simulink model "Copter_System_discrete_sfun"  (Simulink 7.4)
settings: Solver=FixedStepDiscrete  StartTime=0.0  StopTime=tend  FixedStep=Ts  RelTol=1e-3
values from neighbouring files (symbols this model uses):
  f1 = (I_y-I_z)/I_x    [quadrocopter_param.m]
  f2 = rot.J_z/I_x    [quadrocopter_param.m]
  f3 = (I_z-I_x)/I_y    [quadrocopter_param.m]
  f4 = rot.J_z/I_y    [quadrocopter_param.m]
  f5 = (I_x-I_y)/I_z    [quadrocopter_param.m]
  g = 9.81    [complementary_filter_param.m]    (also in quadrocopter_param.m)
  I_x = elec.I_x+bat.I_x+2*boom.I_1x+2*boom.I_1y+2*mot.I_1x+2*mot.I_1y+                             2*rot.I_1x+2*rot.I_1y    [quadrocopter_param.m]
  I_y = elec.I_y+bat.I_y+2*boom.I_1x+2*boom.I_1y+2*mot.I_1x+2*mot.I_1y+                             2*rot.I_1x+2*rot.I_1y    [quadrocopter_param.m]
  I_z = elec.I_z+bat.I_z+4*boom.I_1z+4*mot.I_1z+4*rot.I_1z    [quadrocopter_param.m]
  m = elec.m+bat.m+boom.m+(4*mot.m)+(4*rot.m)    [quadrocopter_param.m]
  shift = 1000    [quadrocopter_param.m]
  speed = rpm.*(2*pi/60)    [quadrocopter_param.m]
  thrust = [0.58 1 1.33 2 2.54 3.33 4.08 4.54]    [quadrocopter_param.m]
  Ts = 0.01    [complementary_filter_param.m]    (also in quadrocopter_param.m)
undefined symbols (not defined in the file or in its folder): boom, DiscIntNeverNeededParam
libraries: simulink x4, dspinverses x1
settings Model: Creator=Sreekanth  LastModifiedBy=Sreekanth
settings DebuggingCC: ArtificialAlgebraicLoopMsg=none

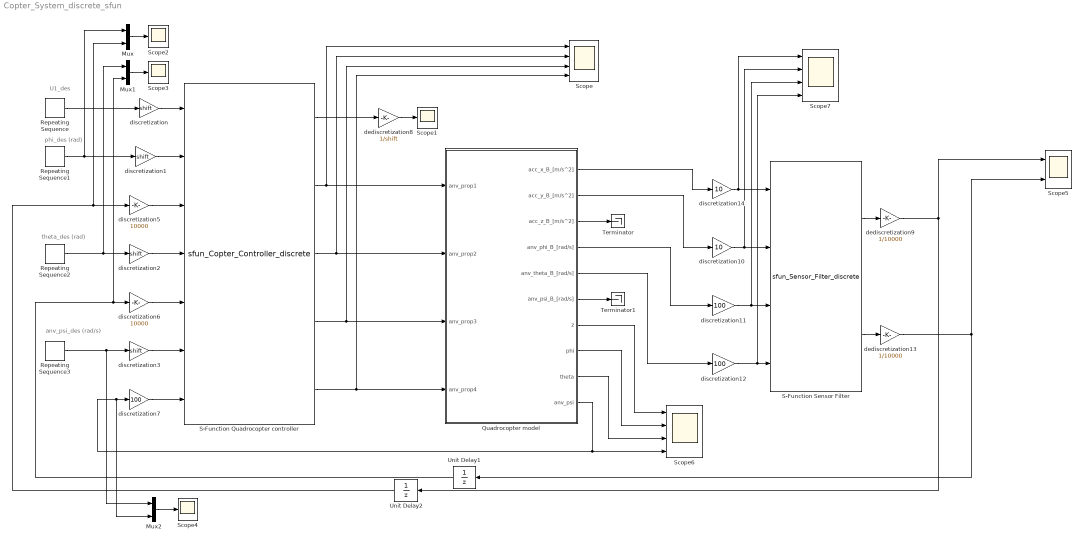
== system Copter_System_discrete_sfun ==
  note: U1_des
  note: phi_des (rad)
  note: theta_des (rad)
  note: anv_psi_des (rad/s)
  Mux : Mux  Inputs=2
  Mux1 : Mux  Inputs=2
  Mux2 : Mux  Inputs=2
  Quadrocopter model : Subsystem
  Repeating Sequence : simulink/Sources/Repeating Sequence  SystemSampleTime=-1  rep_seq_t=desforce.time  rep_seq_y=desforce.force
  Repeating Sequence1 : simulink/Sources/Repeating Sequence  SystemSampleTime=-1  rep_seq_t=desroll.time  rep_seq_y=desroll.angle
  Repeating Sequence2 : simulink/Sources/Repeating Sequence  SystemSampleTime=-1  rep_seq_t=despitch.time  rep_seq_y=despitch.angle
  Repeating Sequence3 : simulink/Sources/Repeating Sequence  SystemSampleTime=-1  rep_seq_t=desyaw.time  rep_seq_y=desyaw.velocity
  S-Function Quadrocopter controller : S-Function  FunctionName=sfun_Copter_Controller_discrete  Parameters=[8 4 8 8 4 8 8 3 1]  EnableBusSupport=off
      mask Display:
      | port_label('input',1,'U1_des')
      | port_label('input',2,'phi_des')
      | port_label('input',3,'phi_filt')
      | port_label('input',4,'theta_des')
      | port_label('input',5,'theta_filt')
      | port_label('input',6,'anv_psi_des')
      | port_label('input',7,'anv_psi')
      | port_label('output',1,'U1_out')
      | port_label('output',2,'anv_prop1')
      | port_label('output',3,'anv_prop2')
      | port_label('output',4,'anv_prop3')
      | port_label('output',5,'anv_prop4')
  S-Function Sensor Filter : S-Function  FunctionName=sfun_Sensor_Filter_discrete  EnableBusSupport=off
      mask Display:
      | port_label('input',1,'acc_x_B')
      | port_label('input',2,'acc_y_B')
      | port_label('input',3,'anv_phi_B')
      | port_label('input',4,'anv_theta_B')
      | port_label('output',1,'phi_filt')
      | port_label('output',2,'theta_filt')
  Scope : Scope  NumInputPorts=4
      settings: TimeRange=30  YMin=0~0~0~0  YMax=6000~6000~6000~6000
  Scope{1..4} (4 alike) : Scope
      Scope1 settings: YMax=20
      Scope2 settings: TimeRange=30  YMin=0  YMax=0.275  SaveName=ScopeData2
      Scope3 settings: TimeRange=30  YMin=0  YMax=0.275  SaveName=ScopeData14
      Scope4 settings: TimeRange=30  YMin=-0.02  YMax=0.3  SaveName=ScopeData15
  Scope5 : Scope  NumInputPorts=2
      settings: YMin=-5~-5  YMax=5~5  SaveName=ScopeData12
  Scope6 : Scope  NumInputPorts=4
      settings: TimeRange=30  YMin=-5~-5~-5~-5  YMax=5~5~5~5  SaveName=ScopeData13
  Scope7 : Scope  NumInputPorts=4
      settings: TimeRange=30  YMin=-5~-5~-5~-5  YMax=5~5~5~5  SaveName=ScopeData16
  Terminator : Terminator
  Terminator1 : Terminator
  Unit Delay1 : UnitDelay  SampleTime=-1
  Unit Delay2 : UnitDelay  SampleTime=-1
  dediscretization13 : Gain  Gain=1/10000  ParameterDataType=fixdt(1, 16)  ParameterScaling=2^0  OutDataTypeMode=double  OutDataType=fixdt(1, 16)  OutScaling=2^0  OutDataTypeStr=double
  dediscretization8 : Gain  Gain=1/shift  ParameterDataType=fixdt(1, 16)  ParameterScaling=2^0  OutDataTypeMode=double  OutDataType=fixdt(1, 16)  OutScaling=2^0  OutDataTypeStr=double
  dediscretization9 : Gain  Gain=1/10000  ParameterDataType=fixdt(1, 16)  ParameterScaling=2^0  OutDataTypeMode=double  OutDataType=fixdt(1, 16)  OutScaling=2^0  OutDataTypeStr=double
  discretization{,1..3} (4 alike) : Gain  Gain=shift  ParameterDataType=fixdt(1, 16)  ParameterScaling=2^0  OutDataTypeMode=int16  OutDataType=fixdt(1, 16)  OutScaling=2^0  OutDataTypeStr=int16
  discretization10 : Gain  Gain=10  ParameterDataType=fixdt(1, 16)  ParameterScaling=2^0  OutDataTypeMode=int16  OutDataType=fixdt(1, 16)  OutScaling=2^0  OutDataTypeStr=int16
  discretization11 : Gain  Gain=100  ParameterDataType=fixdt(1, 16)  ParameterScaling=2^0  OutDataTypeMode=int16  OutDataType=fixdt(1, 16)  OutScaling=2^0  OutDataTypeStr=int16
  discretization12 : Gain  Gain=100  ParameterDataType=fixdt(1, 16)  ParameterScaling=2^0  OutDataTypeMode=int16  OutDataType=fixdt(1, 16)  OutScaling=2^0  OutDataTypeStr=int16
  discretization14 : Gain  Gain=10  ParameterDataType=fixdt(1, 16)  ParameterScaling=2^0  OutDataTypeMode=int16  OutDataType=fixdt(1, 16)  OutScaling=2^0  OutDataTypeStr=int16
  discretization5 : Gain  Gain=10000  ParameterDataType=fixdt(1, 16)  ParameterScaling=2^0  OutDataTypeMode=int16  OutDataType=fixdt(1, 16)  OutScaling=2^0  OutDataTypeStr=int16
  discretization6 : Gain  Gain=10000  ParameterDataType=fixdt(1, 16)  ParameterScaling=2^0  OutDataTypeMode=int16  OutDataType=fixdt(1, 16)  OutScaling=2^0  OutDataTypeStr=int16
  discretization7 : Gain  Gain=100  ParameterDataType=fixdt(1, 16)  ParameterScaling=2^0  OutDataTypeMode=int16  OutDataType=fixdt(1, 16)  OutScaling=2^0  OutDataTypeStr=int16
  wires:
  Repeating Sequence/1 -> discretization/1
  discretization/1 -> S-Function Quadrocopter controller/1
  Repeating Sequence1/1 -> discretization1/1, Mux/1
  discretization1/1 -> S-Function Quadrocopter controller/2
  Repeating Sequence2/1 -> discretization2/1, Mux1/1
  discretization2/1 -> S-Function Quadrocopter controller/4
  Repeating Sequence3/1 -> discretization3/1, Mux2/1
  discretization3/1 -> S-Function Quadrocopter controller/6
  discretization5/1 -> S-Function Quadrocopter controller/3
  discretization6/1 -> S-Function Quadrocopter controller/5
  discretization7/1 -> S-Function Quadrocopter controller/7
  S-Function Quadrocopter controller/1 -> dediscretization8/1
  S-Function Quadrocopter controller/2 -> Scope/1, Quadrocopter model/1(anv_prop1)
  S-Function Quadrocopter controller/3 -> Scope/2, Quadrocopter model/2(anv_prop2)
  S-Function Quadrocopter controller/4 -> Scope/3, Quadrocopter model/3(anv_prop3)
  S-Function Quadrocopter controller/5 -> Scope/4, Quadrocopter model/4(anv_prop4)
  dediscretization8/1 -> Scope1/1
  Quadrocopter model/3(acc_z_B_[m/s^2]) -> Terminator/1
  Quadrocopter model/6(anv_psi_B_[rad/s]) -> Terminator1/1
  discretization14/1 -> S-Function Sensor Filter/1, Scope7/1
  discretization10/1 -> S-Function Sensor Filter/2, Scope7/2
  discretization11/1 -> S-Function Sensor Filter/3, Scope7/3
  discretization12/1 -> S-Function Sensor Filter/4, Scope7/4
  S-Function Sensor Filter/1 -> dediscretization9/1
  S-Function Sensor Filter/2 -> dediscretization13/1
  dediscretization9/1 -> Scope5/1, Unit Delay2/1
  Quadrocopter model/1(acc_x_B_[m/s^2]) -> discretization14/1
  Quadrocopter model/2(acc_y_B_[m/s^2]) -> discretization10/1
  Quadrocopter model/4(anv_phi_B_[rad/s]) -> discretization11/1
  Quadrocopter model/5(anv_theta_B_[rad/s]) -> discretization12/1
  dediscretization13/1 -> Scope5/2, Unit Delay1/1
  Quadrocopter model/10(anv_psi) -> Scope6/4, discretization7/1, Mux2/2
  Unit Delay1/1 -> discretization6/1, Mux1/2
  Unit Delay2/1 -> discretization5/1, Mux/2
  Mux/1 -> Scope2/1
  Mux1/1 -> Scope3/1
  Mux2/1 -> Scope4/1
  Quadrocopter model/7(z) -> Scope6/1
  Quadrocopter model/8(phi) -> Scope6/2
  Quadrocopter model/9(theta) -> Scope6/3

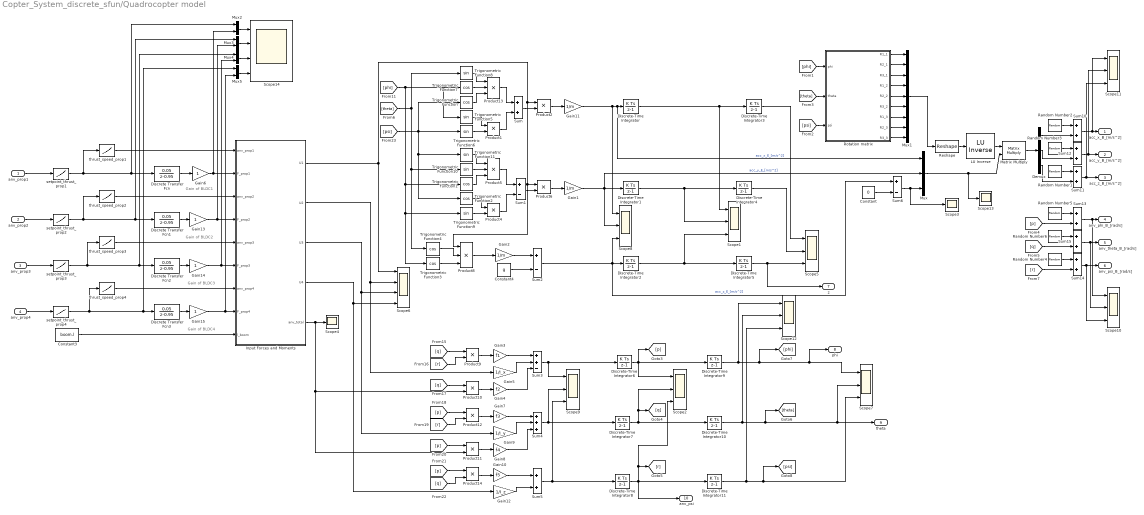
== system Copter_System_discrete_sfun/Quadrocopter model ==
  note: Gain of BLDC1
  note: Gain of BLDC2
  note: Gain of BLDC3
  note: Gain of BLDC4
  anv_prop1 : Inport  OutDataType=fixdt(1, 16)  OutScaling=2^0
  anv_prop2 : Inport  Port=2  OutDataType=fixdt(1, 16)  OutScaling=2^0
  anv_prop3 : Inport  Port=3  OutDataType=fixdt(1, 16)  OutScaling=2^0
  anv_prop4 : Inport  Port=4  OutDataType=fixdt(1, 16)  OutScaling=2^0
  " LU Inverse" : dspinverses/ LU Inverse  SystemSampleTime=-1
  Constant : Constant  Value=0  OutDataType=fixdt(1, 16)  OutScaling=2^0  SampleTime=Ts
  Constant3 : Constant  Value=boom.l  OutDataType=fixdt(1, 16)  OutScaling=2^0
  Constant4 : Constant  Value=g  OutDataType=fixdt(1, 16)  OutScaling=2^0  SampleTime=Ts
  Demux : Demux  Outputs=3
  Discrete Transfer Fcn{,1..3} (4 alike) : DiscreteTransferFcn  Numerator=[0.05]  Denominator=[1 -0.95]  SampleTime=Ts  OutDataTypeStr=int16
  Discrete-Time Integrator{,1..11} (12 alike) : DiscreteIntegrator  SampleTime=Ts  OutDataType=fixdt(1, 16)  OutScaling=2^0  ICPrevOutput=DiscIntNeverNeededParam  ICPrevScaledInput=DiscIntNeverNeededParam
  Gain1 : Gain  Gain=1/m  ParameterDataType=fixdt(1, 16)  ParameterScaling=2^0  OutDataType=fixdt(1, 16)  OutScaling=2^0
  Gain10 : Gain  Gain=f5  ParameterDataType=fixdt(1, 16)  ParameterScaling=2^0  OutDataType=fixdt(1, 16)  OutScaling=2^0
  Gain11 : Gain  Gain=1/m  ParameterDataType=fixdt(1, 16)  ParameterScaling=2^0  OutDataType=fixdt(1, 16)  OutScaling=2^0
  Gain12 : Gain  Gain=1/I_z  ParameterDataType=fixdt(1, 16)  ParameterScaling=2^0  OutDataType=fixdt(1, 16)  OutScaling=2^0
  Gain{6,13..15} (4 alike) : Gain  ParameterDataType=fixdt(1, 16)  ParameterScaling=2^0  OutDataTypeMode=double  OutDataType=fixdt(1, 16)  OutScaling=2^0  OutDataTypeStr=double
  Gain2 : Gain  Gain=1/m  ParameterDataType=fixdt(1, 16)  ParameterScaling=2^0  OutDataType=fixdt(1, 16)  OutScaling=2^0
  Gain3 : Gain  Gain=f1  ParameterDataType=fixdt(1, 16)  ParameterScaling=2^0  OutDataType=fixdt(1, 16)  OutScaling=2^0
  Gain4 : Gain  Gain=f2  ParameterDataType=fixdt(1, 16)  ParameterScaling=2^0  OutDataType=fixdt(1, 16)  OutScaling=2^0
  Gain5 : Gain  Gain=1/I_x  ParameterDataType=fixdt(1, 16)  ParameterScaling=2^0  OutDataType=fixdt(1, 16)  OutScaling=2^0
  Gain7 : Gain  Gain=f3  ParameterDataType=fixdt(1, 16)  ParameterScaling=2^0  OutDataType=fixdt(1, 16)  OutScaling=2^0
  Gain8 : Gain  Gain=f4  ParameterDataType=fixdt(1, 16)  ParameterScaling=2^0  OutDataType=fixdt(1, 16)  OutScaling=2^0
  Gain9 : Gain  Gain=1/I_y  ParameterDataType=fixdt(1, 16)  ParameterScaling=2^0  OutDataType=fixdt(1, 16)  OutScaling=2^0
  Input Forces and Moments : Stateflow chart
  Matrix Multiply : Product  Multiplication=Matrix(*)  OutDataType=sfix(16)  OutScaling=2^0
  Mux : Mux  Inputs=3
  Mux1 : Mux  Inputs=9
  Mux{2..5} (4 alike) : Mux  Inputs=2
  Product{1..2,4,6,9..12,14} (9 alike) : Product  OutDataType=fixdt(1, 16)  OutScaling=2^0  RndMeth=Zero
  Product13 : Product  Inputs=3  OutDataType=fixdt(1, 16)  OutScaling=2^0  RndMeth=Zero
  Product5 : Product  Inputs=3  OutDataType=fixdt(1, 16)  OutScaling=2^0  RndMeth=Zero
  Product8 : Product  Inputs=3  OutDataType=fixdt(1, 16)  OutScaling=2^0  RndMeth=Zero
  Random Number{1..6} (6 alike) : RandomNumber  Variance=0  SampleTime=Ts
  Reshape : Reshape  OutputDimensionality=Customize  OutputDimensions=[3,3]
  Rotation matrix : Stateflow chart
  Scope{1..2,5,7..12} (9 alike) : Scope  NumInputPorts=3
      Scope1 settings: YMin=-5~-5~-5  YMax=5~5~5  SaveName=ScopeData21
      Scope10 settings: YMin=-5~-5~-5  YMax=5~5~5  SaveName=ScopeData9
      Scope11 settings: YMin=-5~-5~-5  YMax=5~5~5  SaveName=ScopeData10
      Scope12 settings: YMin=-5~-5~-5  YMax=5~5~5  SaveName=ScopeData11
      Scope2 settings: YMin=-5~-5~-5  YMax=5~5~5  SaveName=ScopeData24
      Scope5 settings: YMin=-5~-5~-5  YMax=5~5~5  SaveName=ScopeData3
      Scope7 settings: TimeRange=30  YMin=-0.05~-0.2~-0.5  YMax=0.3~0.15~3  SaveName=ScopeData6
      Scope8 settings: TimeRange=30  YMin=-1~-1~3  YMax=1~1~10  SaveName=ScopeData7
      Scope9 settings: YMin=-5~-5~-5  YMax=5~5~5  SaveName=ScopeData8
  Scope13 : Scope
      settings: SaveName=ScopeData22
  Scope14 : Scope  NumInputPorts=4
      settings: YMin=-5~-5~-5~-5  YMax=5~5~5~5  SaveName=ScopeData23
  Scope3 : Scope
      settings: SaveName=ScopeData19
  Scope4 : Scope
      settings: SaveName=ScopeData4
  Scope6 : Scope  NumInputPorts=4
      settings: YMin=-5~-5~-5~-5  YMax=5~5~5~5  SaveName=ScopeData5
  Sum{,5,10..15} (8 alike) : Sum  OutDataType=fixdt(1, 16)  OutScaling=2^0
  Sum1 : Sum  Inputs=+-  OutDataType=fixdt(1, 16)  OutScaling=2^0
  Sum2 : Sum  Inputs=+-  OutDataType=fixdt(1, 16)  OutScaling=2^0
  Sum3 : Sum  Inputs=++-  OutDataType=fixdt(1, 16)  OutScaling=2^0
  Sum4 : Sum  Inputs=+++  OutDataType=fixdt(1, 16)  OutScaling=2^0
  Sum6 : Sum  Inputs=+-  OutDataType=fixdt(1, 16)  OutScaling=2^0
  Trigonometric Function{,1..4,7} (6 alike) : Trigonometry  Operator=cos
  Trigonometric Function{5..6,8..11} (6 alike) : Trigonometry
  setpoint_thrust_prop{1..4} (4 alike) : Lookup  InputValues=[0 40 175]  Table=[0 500 4500]./1000  LookUpMeth=Interpolation-Use End Values  OutDataTypeMode=double  OutDataType=fixdt(1, 16)  OutScaling=2^0  OutDataTypeStr=double
  thrust_speed_prop{1..4} (4 alike) : Lookup  InputValues=thrust  Table=speed  LookUpMeth=Interpolation-Use End Values  OutDataType=fixdt(1, 16)  OutScaling=2^0
  acc_x_B_[m/s^2] : Outport  OutDataType=fixdt(1, 16)  OutScaling=2^0
  acc_y_B_[m/s^2] : Outport  Port=2  OutDataType=fixdt(1, 16)  OutScaling=2^0
  acc_z_B_[m/s^2] : Outport  Port=3  OutDataType=fixdt(1, 16)  OutScaling=2^0
  anv_phi_B_[rad/s] : Outport  Port=4  OutDataType=fixdt(1, 16)  OutScaling=2^0
  anv_theta_B_[rad/s] : Outport  Port=5  OutDataType=fixdt(1, 16)  OutScaling=2^0
  anv_psi_B_[rad/s] : Outport  Port=6  OutDataType=fixdt(1, 16)  OutScaling=2^0
  z : Outport  Port=7  OutDataType=fixdt(1, 16)  OutScaling=2^0
  phi : Outport  Port=8  OutDataType=fixdt(1, 16)  OutScaling=2^0
  theta : Outport  Port=9  OutDataType=fixdt(1, 16)  OutScaling=2^0
  anv_psi : Outport  Port=10  OutDataType=fixdt(1, 16)  OutScaling=2^0
  wires:
  Sum14/1 -> Scope10/3, anv_psi_B_[rad/s]/1
  Sum15/1 -> Scope10/2, anv_theta_B_[rad/s]/1
  Sum13/1 -> Scope10/1, anv_phi_B_[rad/s]/1
  [q] -> Sum15/2
  Random Number6/1 -> Sum15/1
  [r] -> Sum14/2
  Random Number4/1 -> Sum14/1
  [p] -> Sum13/2
  Random Number5/1 -> Sum13/1
  Sum11/1 -> Scope11/3, acc_z_B_[m/s^2]/1
  Sum12/1 -> Scope11/2, acc_y_B_[m/s^2]/1
  Sum10/1 -> Scope11/1, acc_x_B_[m/s^2]/1
  Demux/2 -> Sum12/2
  Random Number3/1 -> Sum12/1
  Demux/3 -> Sum11/2
  Random Number1/1 -> Sum11/1
  Demux/1 -> Sum10/2
  Random Number2/1 -> Sum10/1
  Matrix Multiply/1 -> Demux/1
  anv_prop3/1 -> setpoint_thrust_prop3/1
  anv_prop4/1 -> setpoint_thrust_prop4/1
  Reshape/1 -> " LU Inverse"/1
  Mux/1 -> Matrix Multiply/2, Scope13/1
  Mux1/1 -> Reshape/1
  Rotation matrix/9(R3_3) -> Mux1/9
  Rotation matrix/8(R2_3) -> Mux1/8
  Rotation matrix/7(R1_3) -> Mux1/7
  Rotation matrix/6(R3_2) -> Mux1/6
  Rotation matrix/5(R2_2) -> Mux1/5
  Rotation matrix/4(R1_2) -> Mux1/4
  Rotation matrix/3(R3_1) -> Mux1/3
  Rotation matrix/2(R2_1) -> Mux1/2
  Rotation matrix/1(R1_1) -> Mux1/1
  [psi] -> Rotation matrix/3(psi)
  [theta] -> Rotation matrix/2(theta)
  [phi] -> Rotation matrix/1(phi)
  anv_prop2/1 -> setpoint_thrust_prop2/1
  anv_prop1/1 -> setpoint_thrust_prop1/1
  Constant4/1 -> Sum2/2
  Trigonometric Function4/1 -> Product8/2
  Trigonometric Function3/1 -> Product8/3
  Gain2/1 -> Sum2/1
  Gain11/1 -> Scope8/1, Discrete-Time Integrator/1, Mux/1  "acc_x_E_[m/s^2]"
  Product6/1 -> Gain1/1
  Sum1/1 -> Product6/2
  Product5/1 -> Sum1/1
  Trigonometric Function1/1 -> Product5/3
  Trigonometric Function10/1 -> Product5/2
  Trigonometric Function11/1 -> Product5/1
  Product4/1 -> Sum1/2
  Trigonometric Function2/1 -> Product4/1
  Trigonometric Function9/1 -> Product4/2
  Product2/1 -> Gain11/1
  Sum/1 -> Product2/2
  Product13/1 -> Sum/1
  Trigonometric Function/1 -> Product13/3
  Trigonometric Function7/1 -> Product13/2
  Trigonometric Function8/1 -> Product13/1
  Product1/1 -> Sum/2
  Trigonometric Function5/1 -> Product1/1
  Trigonometric Function6/1 -> Product1/2
  [psi] -> Trigonometric Function2/1, Trigonometric Function11/1, Trigonometric Function/1, Trigonometric Function6/1
  Discrete-Time Integrator/1 -> Scope1/1, Discrete-Time Integrator3/1
  Discrete-Time Integrator1/1 -> Scope1/2, Discrete-Time Integrator4/1
  Discrete-Time Integrator2/1 -> Scope1/3, Discrete-Time Integrator5/1
  [theta] -> Trigonometric Function10/1, Trigonometric Function4/1, Trigonometric Function8/1
  Gain1/1 -> Scope8/2, Discrete-Time Integrator1/1, Mux/2  "acc_y_E_[m/s^2]"
  [phi] -> Trigonometric Function9/1, Trigonometric Function3/1, Trigonometric Function1/1, Trigonometric Function7/1, Trigonometric Function5/1
  Product8/1 -> Gain2/1
  Sum2/1 -> Scope8/3, Discrete-Time Integrator2/1, Sum6/1  "acc_z_E_[m/s^2]"
  Discrete-Time Integrator3/1 -> Scope5/1
  Discrete-Time Integrator4/1 -> Scope5/2
  Discrete-Time Integrator5/1 -> Scope5/3, z/1
  Constant3/1 -> Input Forces and Moments/9(l_boom)
  Sum5/1 -> Scope9/3, Discrete-Time Integrator8/1
  Input Forces and Moments/4(U4) -> Scope6/4, Gain12/1
  Gain12/1 -> Sum5/2
  Gain10/1 -> Sum5/1
  Product14/1 -> Gain10/1
  [q] -> Product14/2
  [p] -> Product14/1
  Sum4/1 -> Scope9/2, Discrete-Time Integrator7/1
  Input Forces and Moments/3(U3) -> Scope6/3, Gain9/1
  Gain8/1 -> Sum4/3
  Gain9/1 -> Sum4/2
  Product11/1 -> Gain8/1
  [p] -> Product11/1
  Gain7/1 -> Sum4/1
  Product12/1 -> Gain7/1
  [r] -> Product12/2
  [p] -> Product12/1
  Input Forces and Moments/1(U1) -> Product8/1, Product6/1, Product2/1, Scope6/1
  Sum3/1 -> Scope9/1, Discrete-Time Integrator6/1
  Gain4/1 -> Sum3/3
  Gain5/1 -> Sum3/2
  Input Forces and Moments/2(U2) -> Scope6/2, Gain5/1
  Product10/1 -> Gain4/1
  [q] -> Product10/1
  Gain3/1 -> Sum3/1
  Product9/1 -> Gain3/1
  [r] -> Product9/2
  [q] -> Product9/1
  Input Forces and Moments/5(anv_total) -> Product11/2, Product10/2, Scope4/1
  Discrete-Time Integrator9/1 -> Scope12/1, [phi], Scope7/1, phi/1
  Discrete-Time Integrator10/1 -> Scope12/2, [theta], Scope7/2, theta/1
  Discrete-Time Integrator11/1 -> Scope12/3, Scope7/3, [psi]
  Discrete-Time Integrator6/1 -> Scope2/1, [p], Discrete-Time Integrator9/1
  Discrete-Time Integrator7/1 -> Scope2/2, [q], Discrete-Time Integrator10/1
  Discrete-Time Integrator8/1 -> Scope2/3, [r], anv_psi/1, Discrete-Time Integrator11/1
  Constant/1 -> Sum6/2
  Sum6/1 -> Mux/3, Scope3/1
  " LU Inverse"/1 -> Matrix Multiply/1
  Discrete Transfer Fcn/1 -> Gain6/1
  Discrete Transfer Fcn1/1 -> Gain13/1
  Discrete Transfer Fcn2/1 -> Gain14/1
  Discrete Transfer Fcn3/1 -> Gain15/1
  Mux2/1 -> Scope14/1
  Gain6/1 -> Input Forces and Moments/2(F_prop1), Mux2/2
  Gain13/1 -> Input Forces and Moments/4(F_prop2), Mux3/2
  Gain14/1 -> Input Forces and Moments/6(F_prop3), Mux4/2
  Gain15/1 -> Input Forces and Moments/8(F_prop4), Mux5/2
  Mux3/1 -> Scope14/2
  Mux4/1 -> Scope14/3
  Mux5/1 -> Scope14/4
  thrust_speed_prop1/1 -> Input Forces and Moments/1(anv_prop1)
  thrust_speed_prop3/1 -> Input Forces and Moments/5(anv_prop3)
  thrust_speed_prop4/1 -> Input Forces and Moments/7(anv_prop4)
  thrust_speed_prop2/1 -> Input Forces and Moments/3(anv_prop2)
  setpoint_thrust_prop1/1 -> thrust_speed_prop1/1, Mux2/1, Discrete Transfer Fcn/1
  setpoint_thrust_prop2/1 -> thrust_speed_prop2/1, Discrete Transfer Fcn1/1, Mux3/1
  setpoint_thrust_prop3/1 -> thrust_speed_prop3/1, Discrete Transfer Fcn2/1, Mux4/1
  setpoint_thrust_prop4/1 -> thrust_speed_prop4/1, Discrete Transfer Fcn3/1, Mux5/1

== matlab function Quadrocopter model/Input Forces and Moments ==
  data: anv_prop1 input double; F_prop1 input double; anv_prop2 input double; F_prop2 input double; anv_prop3 input double; F_prop3 input double; anv_prop4 input double; U1 output double; F_prop4 input double; U2 output double; U3 output double; U4 output double; l_boom input double; anv_total output double
function [U1, U2, U3, U4, anv_total] = input(anv_prop1,F_prop1,anv_prop2,...
    F_prop2,anv_prop3,F_prop3,anv_prop4,F_prop4,l_boom)
%#eml

% Calculating Thrust in z-axis with respect to body fixed coordinate system
U1 = F_prop1 + F_prop2 + F_prop3 + F_prop4;             % [N]

% Calculating Torque around x-axis (Roll) due to Thrust
U2 = l_boom*(-F_prop4+F_prop2);                         % [Nm]

% Calculating Torque around y-axis (Pitch) due to Thrust
U3 = l_boom*(-F_prop1+F_prop3);                         % [Nm]

% Calculating Torque around z-axis (Yaw) due to Thrust
U4 = l_boom*(F_prop1-F_prop2+F_prop3-F_prop4);          % [Nm]

% Overall propeller speed
anv_total = anv_prop1-anv_prop2+anv_prop3-anv_prop4;    % [rad/s]

== matlab function Quadrocopter model/Rotation matrix ==
  data: phi input double; theta input double; psi input double; R1_1 output double; R2_1 output double; R3_1 output double; R1_2 output double; R2_2 output double; R3_2 output double; R1_3 output double; R2_3 output double; R3_3 output double
function [ R1_1, R2_1, R3_1, R1_2, R2_2, R3_2, R1_3, R2_3, R3_3] = input...
                                                    (phi, theta, psi)
% Transformation of E-frame to B-Frame
R1_1 = cos(psi)*cos(theta);
R2_1 = sin(psi)*cos(theta);
R3_1 = -sin(theta);
R1_2 = -sin(psi)*cos(phi)+cos(psi)*sin(theta)*sin(phi);
R2_2 = cos(psi)*cos(phi)+sin(psi)*sin(theta)*sin(phi);
R3_2 = cos(theta)*sin(phi);
R1_3 = sin(psi)*sin(phi)+cos(psi)*sin(theta)*cos(phi);
R2_3 = -cos(psi)*sin(phi)+sin(psi)*sin(theta)*cos(phi);
R3_3 = cos(theta)*cos(phi);
